simulink model "QuadModel"  (R2022b)
settings: Solver=VariableStepAuto  StartTime=0.0  StopTime=50  RelTol=1e-3  AbsTol=1e-3  EnableMultiTasking=on
values from neighbouring files (symbols this model uses):
  Ixx = 0.0032    [DroneParameters.mat]
  Iyy = 0.00319347    [DroneParameters.mat]
  Izz = 0.01737    [DroneParameters.mat]
  k = 7.075135827e-05    [DroneParameters.mat]
  mass = 0.28848668    [DroneParameters.mat]
  prD = 6000    [DroneParameters.mat]
  prI = 500    [DroneParameters.mat]
  prP = 2500    [DroneParameters.mat]
  zD = 7500    [DroneParameters.mat]
  zI = 10000    [DroneParameters.mat]
  zP = 25000    [DroneParameters.mat]
undefined symbols (not defined in the file or in its folder): X, Y, Z
libraries: sm_lib x42, nesl_utility x35, slpidlib x4
(part 3 of 3)

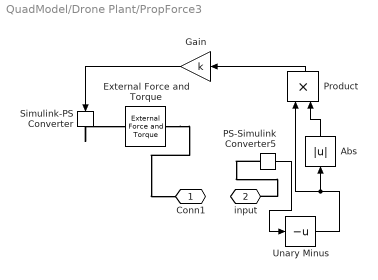
== system QuadModel/Drone Plant/PropForce3 ==
  Abs : Abs  SaturateOnIntegerOverflow=off
  External Force and Torque : sm_lib/Forces and Torques/External Force and Torque  ForceResolutionFrame=AttachedFrame  EnableForceX=off  EnableForceY=off  EnableForceZ=on  EnableForce=off  TorqueResolutionFrame=AttachedFrame  EnableTorqueX=off  EnableTorqueY=off  EnableTorqueZ=off  EnableTorque=off
  Gain : Gain  Gain=k
  PS-Simulink Converter5 : nesl_utility/PS-Simulink Converter  PhysicalDomain=network_engine_domain  SubClassName=ps_output  LeftPortType=input  RightPortType=output  PseudoPeriodic=off  Frequencies=[]  VectorFormat=inherit  Unit=inherit  AffineConversion=off
  Product : Product
  Simulink-PS Converter : nesl_utility/Simulink-PS Converter  PhysicalDomain=network_engine_domain  SubClassName=ps_input  LeftPortType=input  RightPortType=output  PseudoPeriodic=off  Frequencies=[]  NoiseDistribution=none  NoiseParameters=[]  Unit=1  AffineConversion=off  FilteringAndDerivatives=provide  SimscapeFilterOrder=1  InputFilterTimeConstant=0.001  UdotUserProvided=0
  Unary Minus : UnaryMinus
  Conn1 : PMIOPort  Side=Right
  input : PMIOPort  Port=2  Side=Left
  wires:
  Product/1 -> Gain/1
  Abs/1 -> Product/2
  Gain/1 -> Simulink-PS Converter/1
  PS-Simulink Converter5/1 -> Unary Minus/1
  Unary Minus/1 -> Abs/1, Product/1
  connections:
  PS-Simulink Converter5/LConn1 -- input/RConn1
  Simulink-PS Converter/RConn1 -- External Force and Torque/LConn1
  External Force and Torque/RConn1 -- Conn1/RConn1

== matlab function QuadModel/Drone Plant/MATLAB Function ==
  data: u input; alpha output
function alpha = fcn(u)

alpha = 180*u(2)/pi;

== matlab function QuadModel/Drone Plant/MATLAB Function2 ==
  data: u input; gamma output
function gamma = fcn(u)

gamma = 180*u(1)/pi;

== matlab function QuadModel/Drone Plant/MATLAB Function1 ==
  data: u input; beta output
function beta = fcn(u)

beta = 180*u(2)/pi;
